simulink model "mod4"  (R2018b)
settings: Solver=FixedStepAuto  StartTime=0.0  StopTime=400  FixedStep=1e-2  RelTol=1e-3  EnableMultiTasking=on
values from neighbouring files (symbols this model uses):
  d = 0.5    [mod1s.m]
  h = 4    [mod1s.m]
  K = 19    [mod1s.m]
  k1 = 3    [mod1s.m]
  k2 = 40    [mod1s.m]
  T = 29    [mod1s.m]
settings Model: Creator=user  LastModifiedBy=ogure
settings SolverCC: SolverResetMethod=Robust
settings DataIOCC: LimitDataPoints=on  SaveFormat=Array  SaveOutput=off  OutputSaveName=X,X4,L,H
settings OptimizationCC: LifeSpan=inf
settings DebuggingCC: SolverPrmCheckMsg=warning  SFUnexpectedBacktrackingDiag=warning  SFNoUnconditionalDefaultTransitionDiag=warning  SFExecutionAtInitializationDiag=none
settings HardwareCC: ProdBitPerPointer=32  ProdBitPerSizeT=32  ProdBitPerPtrDiffT=32  ProdLargestAtomicFloat=None  ProdIntDivRoundTo=Undefined  ProdEndianess=Unspecified  ProdWordSize=32  ProdHWDeviceType=32-bit Generic
settings ModelReferenceCC: PropagateSignalLabelsOutOfModel=off
settings SFSimCC: SimUseLocalCustomCode=off
settings RTWCC: RTWUseLocalCustomCode=off
settings CodeAppCC: StateflowObjectComments=on
settings GRTTargetCC: TargetLangStandard=C89/C90 (ANSI)  GeneratePreprocessorConditionals=Disable all
settings ConfigComp: CovMetricSettings=dw  CovHtmlReporting=on  CovSaveCumulativeToWorkspaceVar=on  CovSaveSingleToWorkspaceVar=on  CovExternalEMLEnable=off  CovSFcnEnable=off

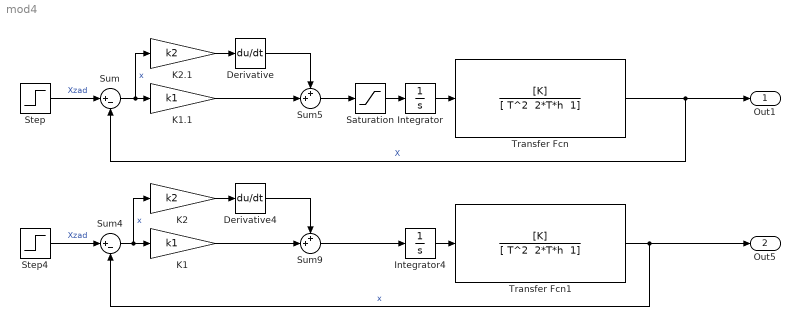
== system mod4 ==
  Derivative : Derivative  CoefficientInTFapproximation=0.00000001
  Derivative4 : Derivative  CoefficientInTFapproximation=0.00000001
  Integrator : Integrator
  Integrator4 : Integrator
  K1 : Gain  Gain=k1
  K1.1 : Gain  Gain=k1
  K2 : Gain  Gain=k2
  K2.1 : Gain  Gain=k2
  Saturation : Saturate  UpperLimit=d  LowerLimit=-d
  Step : Step  Time=0  SampleTime=0
  Step4 : Step  Time=0  SampleTime=0
  Sum : Sum  Inputs=|+-
  Sum4 : Sum  Inputs=|+-
  Sum5 : Sum  Inputs=++|
  Sum9 : Sum  Inputs=++|
  Transfer Fcn : TransferFcn  Numerator=[K]  Denominator="[ T^2  2*T*h  1]"
  Transfer Fcn1 : TransferFcn  Numerator=[K]  Denominator="[ T^2  2*T*h  1]"
  Out1 : Outport  SignalName=x
  Out5 : Outport  Port=2  SignalName=x
  wires:
  Saturation/1 -> Integrator/1
  Transfer Fcn/1 -> Sum/2, Out1/1  "X"
  Integrator/1 -> Transfer Fcn/1
  Sum/1 -> K2.1/1, K1.1/1  "x"
  Step4/1 -> Sum4/1  "Xzad"
  Integrator4/1 -> Transfer Fcn1/1
  Sum9/1 -> Integrator4/1
  Transfer Fcn1/1 -> Out5/1, Sum4/2  "x"
  Step/1 -> Sum/1  "Xzad"
  K1.1/1 -> Sum5/2
  Sum5/1 -> Saturation/1
  K2.1/1 -> Derivative/1
  Derivative/1 -> Sum5/1
  Derivative4/1 -> Sum9/1
  K2/1 -> Derivative4/1
  Sum4/1 -> K2/1, K1/1  "x"
  K1/1 -> Sum9/2
